simulink subsystem "InvertedPendulum"  (R2023a)
settings: Solver=VariableStepAuto  StartTime=0.0  StopTime=10.0  RelTol=1e-3
undefined symbols (not defined in the file): g, l
settings Model: Creator=MY PC  LastModifiedBy=MY PC

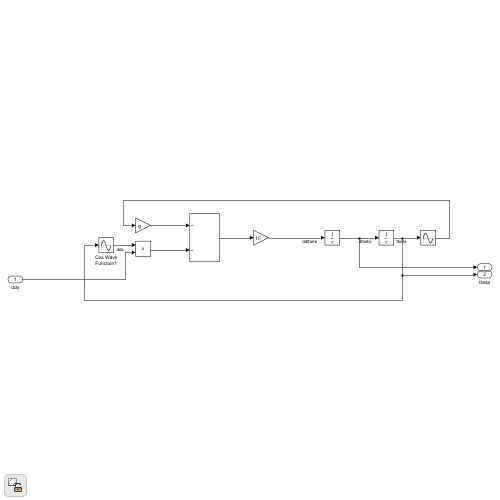
[thumbnail: Simulink's stored preview of the top-level diagram]
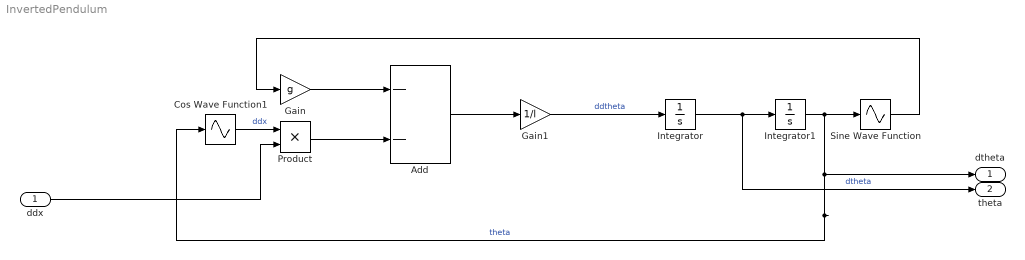
== system InvertedPendulum ==
  ddx : Inport
  Add : Sum  Inputs=--
  Cos Wave Function1 : Sin  TimeSource=Use external signal  Phase=pi/2  SampleTime=0
  Gain : Gain  Gain=g
  Gain1 : Gain  Gain=1/l
  Integrator : Integrator
  Integrator1 : Integrator  InitialCondition=0.9*pi
  Product : Product
  Sine Wave Function : Sin  TimeSource=Use external signal  SampleTime=0
  dtheta : Outport
  theta : Outport  Port=2
  wires:
  Integrator1/1 -> Sine Wave Function/1, Cos Wave Function1/1, dtheta/1  "theta"
  Gain1/1 -> Integrator/1  "ddtheta"
  Gain/1 -> Add/1
  Add/1 -> Gain1/1
  Integrator/1 -> Integrator1/1, theta/1  "dtheta"
  Cos Wave Function1/1 -> Product/1  "ddx"
  Sine Wave Function/1 -> Gain/1
  Product/1 -> Add/2
  ddx/1 -> Product/2
